simulink model "switch_example"  (Simulink 8.5)
settings: Solver=ode45  StartTime=0.0  StopTime=10.0  RelTol=1e-3
libraries: simulink x1
settings Model: Creator=mfoglema  LastModifiedBy=Aranya Dan
settings OptimizationCC: ExpressionDepthLimit=128  InitFltsAndDblsToZero=on
settings DebuggingCC: SaveWithParameterizedLinksMsg=none  SignalResolutionControl=TryResolveAllWithWarning  SolverPrmCheckMsg=warning  MultiTaskDSMMsg=warning  MultiTaskCondExecSysMsg=none  FcnCallInpInsideContextMsg=UseLocalSettings  StateNameClashWarn=none  StrictBusMsg=Warning
settings GRTTargetCC: TargetFcnLib=ansi_tfl_tmw.mat

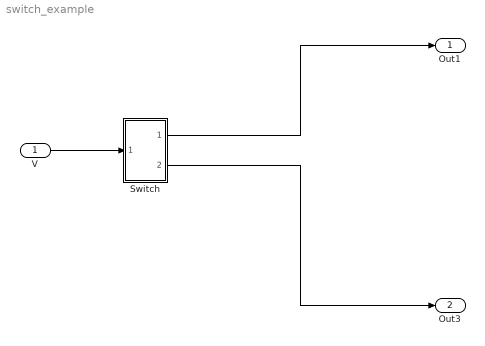
== system switch_example ==
  V : Inport
  Switch : Subsystem
  Out1 : Outport
  Out3 : Outport  Port=2
  wires:
  Switch/1(Out1) -> Out1/1
  Switch/2(Out2) -> Out3/1
  V/1 -> Switch/1(In1)

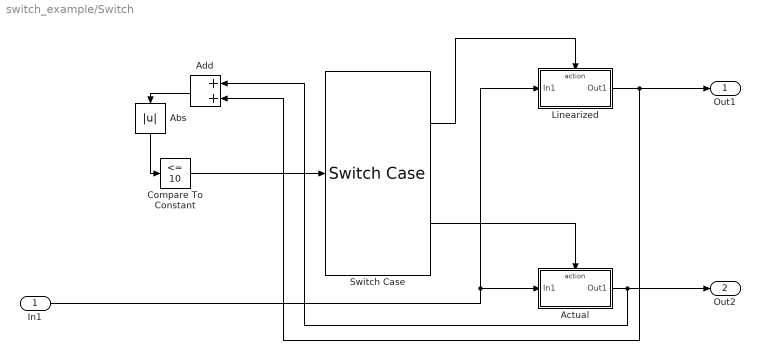
== system switch_example/Switch ==
  In1 : Inport
  Abs : Abs
  Actual : Subsystem  TreatAsAtomicUnit=on
  Add : Sum
  Compare To Constant : simulink/Logic and Bit Operations/Compare To Constant  relop=<=  const=10  OutDataTypeStr=boolean
  Linearized : Subsystem  TreatAsAtomicUnit=on
  Switch Case : SwitchCase  CaseConditions={1,}
  Out1 : Outport
  Out2 : Outport  Port=2
  wires:
  Add/1 -> Abs/1
  Compare To Constant/1 -> Switch Case/1
  Actual/1(Out1) -> Out2/1, Add/1
  In1/1 -> Linearized/1(In1), Actual/1(In1)
  Switch Case/2 -> Actual/Action
  Switch Case/1 -> Linearized/Action
  Linearized/1(Out1) -> Out1/1, Add/2
  Abs/1 -> Compare To Constant/1

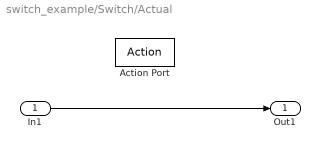
== system switch_example/Switch/Actual ==
  In1 : Inport
  Action Port : ActionPort  ActionType=default
  Out1 : Outport
  wires:
  In1/1 -> Out1/1

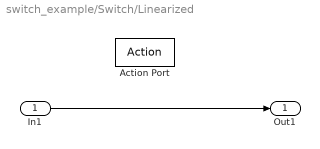
== system switch_example/Switch/Linearized ==
  In1 : Inport
  Action Port : ActionPort  ActionType=case
  Out1 : Outport
  wires:
  In1/1 -> Out1/1
